simulink model "MEC_R2016b"  (R2016b)
settings: Solver=VariableStepAuto  StartTime=0.0  StopTime=40  RelTol=1e-3
undefined symbols (not defined in the file): Ad, Am, Ap, Bd, Bm, Bp, Bw, Cd, Cm, Cp, Dd, Dw
settings Model: Creator=89yos  LastModifiedBy=Yoshida Ryuichiro
settings DataIOCC: ReturnWorkspaceOutputs=on
settings SFSimCC: SimUseLocalCustomCode=on
settings RTWCC: RTWUseLocalCustomCode=on

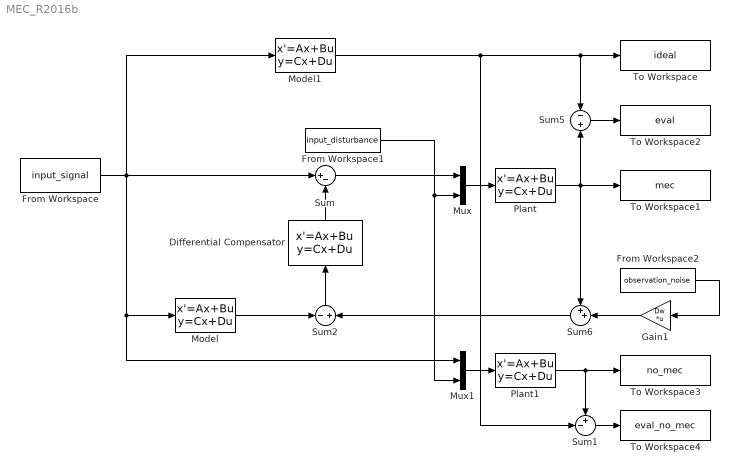
== system MEC_R2016b ==
  Differential Compensator : StateSpace  A=Ad  B=Bd  C=Cd  D=Dd  X0=0
  From Workspace : FromWorkspace  VariableName=input_signal  SampleTime=0
  From Workspace1 : FromWorkspace  VariableName=input_disturbance  SampleTime=0
  From Workspace2 : FromWorkspace  VariableName=observation_noise  SampleTime=0
  Gain1 : Gain  Gain=Dw  Multiplication=Matrix(K*u)
  Model : StateSpace  A=Am  B=Bm  C=Cm  D=zeros(size(Cm,1),size(Bm,2))  X0=0
  Model1 : StateSpace  A=Am  B=Bm  C=Cm  D=zeros(size(Cm,1),size(Bm,2))  X0=0
  Mux : Mux  Inputs=2
  Mux1 : Mux  Inputs=2
  Plant : StateSpace  A=Ap  B=[Bp Bw]  C=Cp  D=zeros(size(Cp,1),size([Bp Bw],2))  X0=0
  Plant1 : StateSpace  A=Ap  B=[Bp Bw]  C=Cp  D=zeros(size(Cp,1),size([Bp Bw],2))  X0=0
  Sum : Sum  Inputs=|+-
  Sum1 : Sum  Inputs=+-|
  Sum2 : Sum  Inputs=-+
  Sum5 : Sum  Inputs=-|+
  Sum6 : Sum  Inputs=++|
  To Workspace : ToWorkspace  VariableName=ideal  SaveFormat=Timeseries  SampleTime=-1
  To Workspace1 : ToWorkspace  VariableName=mec  SaveFormat=Timeseries  SampleTime=-1
  To Workspace2 : ToWorkspace  VariableName=eval  SaveFormat=Timeseries  SampleTime=-1
  To Workspace3 : ToWorkspace  VariableName=no_mec  SaveFormat=Timeseries  SampleTime=-1
  To Workspace4 : ToWorkspace  VariableName=eval_no_mec  SaveFormat=Timeseries  SampleTime=-1
  wires:
  Differential Compensator/1 -> Sum/2
  Sum/1 -> Mux/1
  Model/1 -> Sum2/1
  Sum2/1 -> Differential Compensator/1
  Plant/1 -> Sum5/2, To Workspace1/1, Sum6/1
  From Workspace/1 -> Mux1/1, Model/1, Model1/1, Sum/1
  Mux/1 -> Plant/1
  From Workspace2/1 -> Gain1/1
  Sum5/1 -> To Workspace2/1
  Model1/1 -> Sum1/2, Sum5/1, To Workspace/1
  Gain1/1 -> Sum6/2
  Sum6/1 -> Sum2/2
  From Workspace1/1 -> Mux/2, Mux1/2
  Mux1/1 -> Plant1/1
  Plant1/1 -> Sum1/1, To Workspace3/1
  Sum1/1 -> To Workspace4/1
